simulink model "Galvo_sys_Cdisc_Pcont_cc_nosub_GUT_v63_quantizizer"  (R2013a)
settings: Solver=ode23  StartTime=0.0  StopTime=5e-3  FixedStep=FS  MaxStep=1e-4  RelTol=1e-3
PreLoadFcn:
  | vname=@(x) inputname(1);
  | paramCtrl=evalin('base','paramCtrl;');
  | I_LIM=str2num(paramCtrl.I_LIM);
  | Kbc=str2num(paramCtrl.Kbc);
  | FS=evalin('base','FS;');
InitFcn:
  | %%%%%%  set scope time range
  | T_STOP=str2num(get_param(gcs,'StopTime'));
  | if numel(T_STOP) > 1
  |    T_STOP=T_STOP(2);
  | else
  |    T_STOP=T_STOP(1);
  | end
  | T_STOP=num2str(T_STOP);
  | 
  | %%%%%%  set scope time range in system @init_callback_fct
  | T_STOP=num2str(str2num(get_param(gcs,'StopTime')));
  | 
  | childs = allchild(0);
  | sol=strfind(upper(get(allchild(0),'Tag')),'VIEWER_PARAMETERS');
  | 
  | if iscell(sol)
  |    ind=find(~cellfun(@isempty, strfind(upper(get(allchild(0),'Tag')),'VIEWER_PARAMETERS')));
  | else
  |    ind=sol;
  | end
  | %ind=find(~cellfun(@isempty, {strfind(upper(get(allchild(0),'Tag')),'VIEWER_PARAMETERS'),[]}))
  | if ~isempty(ind)
  |    for k=1:length(childs(ind))
  |       set_param(getfield(get(childs(ind(k)),'UserData'),'block'),'TimeRange',T_STOP);
  |       get_param(getfield(get(childs(ind(k)),'UserData'),'block'),'TimeRange');
  | %    set_param(getfield(get(childs(ind),'UserData'),'block'),'TimeRange',T_STOP);
  | %    get_param(getfield(get(childs(ind),'UserData'),'block'),'TimeRange');
  |    end
  | else
  |     warning(sprintf('VIEWER_PARAMETERS object not found\nOpen the config dialog by hand for the first sim start'))
  | end
StartFcn:
  | I_LIM=str2num(paramCtrl.I_LIM);
  | Kbc=str2num(paramCtrl.Kbc);
  | %FS=evalin('base','FS;');
undefined symbols (not defined in the file or in its folder): FB_EN, JR, KBM, KFR, KMT, KTB, Lc, Rc, Rsh
libraries: simulink x3, simulink_extras x1, dspsigops x1
settings Model: BufferReuse=off  Creator=mainster  LastModifiedBy=mainster
settings SolverCC: AutoInsertRateTranBlk=on
settings DataIOCC: LimitDataPoints=off  SaveOutput=off  SaveTime=off
settings OptimizationCC: BlockReduction=off  OptimizeBlockIOStorage=off  BufferReuse=off  ExpressionFolding=off  LocalBlockOutputs=off
settings ModelReferenceCC: ModelReferenceNumInstancesAllowed=Single

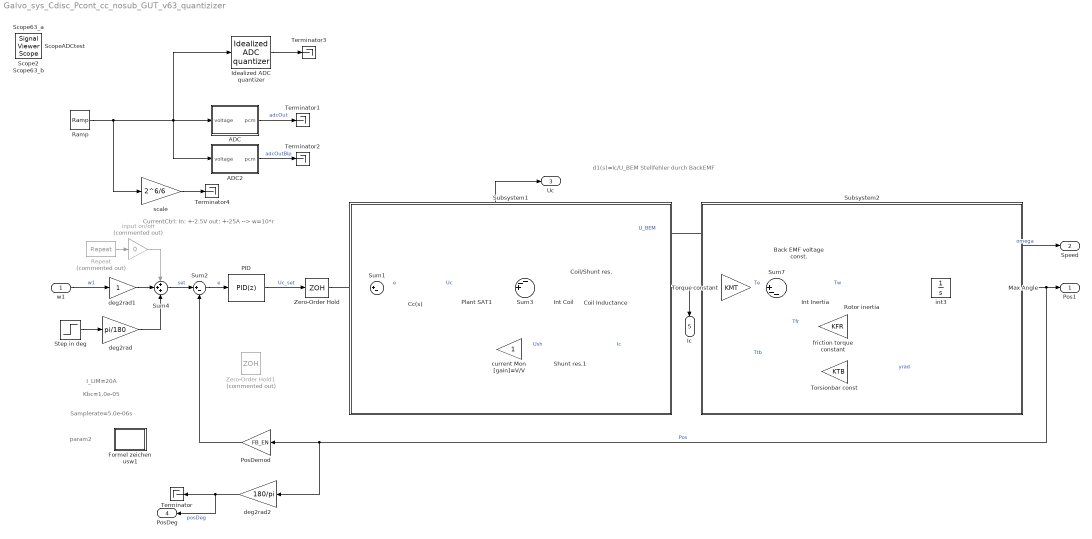
== system Galvo_sys_Cdisc_Pcont_cc_nosub_GUT_v63_quantizizer ==
  note: I_LIM=20A
  note: Kbc=1.0e-05
  note: Samplerate=5.0e-06s
  note: d1(s)=Ic/U_BEM
      | Stellfehler durch BackEMF
  note: param2
  note: CurrentCtrl:
      | In:		+-2.5V
      | out: 	+-25A
      | --> w=10*r
  w1 : Inport
  ADC : Subsystem
      mask Display: fprintf('ADC\n4-bit\n0-3V');
  ADC2 : Subsystem
      mask Display: fprintf('ADC\n4-bit\n-3...+3V');
  Back EMF voltage const. : Gain  Gain=KBM
  Cc(s) : simulink/Continuous/PID Controller  Controller=P  TimeDomain=Continuous-time  SampleTime=-1  IntegratorMethod=Forward Euler  FilterMethod=Forward Euler  Form=Ideal  P=18.7463154861029  I=14078.2261040339  D=0  N=100  InitialConditionSource=internal  InitialConditionForIntegrator=0  InitialConditionForFilter=0  ExternalReset=none  LimitOutput=off  UpperSaturationLimit=inf  LowerSaturationLimit=-inf  LinearizeAsGain=on  AntiWindupMode=none  Kb=1  TrackingMode=off  Kt=1  PParamMin=[]  PParamMax=[]  IParamMin=[]  IParamMax=[]  DParamMin=[]  DParamMax=[]  NParamMin=[]  NParamMax=[]  KbParamMin=[]  KbParamMax=[]  KtParamMin=[]  KtParamMax=[]  POutMin=[]  POutMax=[]  IOutMin=[]  IOutMax=[]  DOutMin=[]  DOutMax=[]  NOutMin=[]  NOutMax=[]  KbOutMin=[]  KbOutMax=[]  KtOutMin=[]  KtOutMax=[]  IntegratorOutMin=[]  IntegratorOutMax=[]  FilterOutMin=[]  FilterOutMax=[]  SumOutMin=[]  SumOutMax=[]  SumI1OutMin=[]  SumI1OutMax=[]  SumI2OutMin=[]  SumI2OutMax=[]  SumI3OutMin=[]  SumI3OutMax=[]  SumDOutMin=[]  SumDOutMax=[]  SaturationOutMin=[]  SaturationOutMax=[]  IntegratorContinuousStateAttributes=''  IntegratorStateMustResolveToSignalObject=off  IntegratorRTWStateStorageClass=Auto  FilterContinuousStateAttributes=''  FilterStateMustResolveToSignalObject=off  FilterRTWStateStorageClass=Auto
  Coil Inductance : Gain  Gain=1/Lc
  Coil/Shunt res. : Gain  Gain=Rc+Rsh
  Formel zeichen usw1 : Subsystem
  Idealized ADC quantizer : simulink_extras/Additional Discrete/Idealized ADC quantizer  NumberOfConverterBits=6  Vmin=-3  Vmax=3  OutputDataType=int16  OutputNegativeValues=on
  Int Coil : Integrator
  Int Inertia : Integrator
  Max Angle : Saturate  UpperLimit=20*pi/180  LowerLimit=-20*pi/180
      settings: AttributesFormatString=Max=%<UpperLimit>\nMin=%<LowerLimit>
  PID : simulink/Continuous/PID Controller  Controller=PID  TimeDomain=Discrete-time  SampleTime=FS  IntegratorMethod=Forward Euler  FilterMethod=Forward Euler  Form=Parallel  P=0.563018062290823  I=5.34105790707236  D=0.011981641194752  N=2584.7602075578  InitialConditionSource=internal  InitialConditionForIntegrator=0  InitialConditionForFilter=0  ExternalReset=none  IgnoreLimit=on  LimitOutput=on  UpperSaturationLimit=30  LowerSaturationLimit=-30  LinearizeAsGain=off  AntiWindupMode=clamping  Kb=0.1  TrackingMode=off  Kt=0  PParamMin=[]  PParamMax=[]  IParamMin=[]  IParamMax=[]  DParamMin=[]  DParamMax=[]  NParamMin=[]  NParamMax=[]  KbParamMin=[]  KbParamMax=[]  KtParamMin=[]  KtParamMax=[]  POutMin=[]  POutMax=[]  IOutMin=[]  IOutMax=[]  DOutMin=[]  DOutMax=[]  NOutMin=[]  NOutMax=[]  KbOutMin=[]  KbOutMax=[]  KtOutMin=[]  KtOutMax=[]  IntegratorOutMin=[]  IntegratorOutMax=[]  FilterOutMin=[]  FilterOutMax=[]  SumOutMin=[]  SumOutMax=[]  SumI1OutMin=[]  SumI1OutMax=[]  SumI2OutMin=[]  SumI2OutMax=[]  SumI3OutMin=[]  SumI3OutMax=[]  SumDOutMin=[]  SumDOutMax=[]  SaturationOutMin=[]  SaturationOutMax=[]  IntegratorContinuousStateAttributes=''  IntegratorStateMustResolveToSignalObject=off  IntegratorRTWStateStorageClass=Auto  FilterContinuousStateAttributes=''  FilterStateMustResolveToSignalObject=off  FilterRTWStateStorageClass=Auto
  Plant SAT1 : Saturate  UpperLimit=30  LowerLimit=-30
      settings: AttributesFormatString=U_lim=+-%<UpperLimit>V
  PosDemod : Gain  Gain=FB_EN
  Ramp : simulink/Sources/Ramp  slope=6/5e-3  start=0  X0=-3
  Repeat : dspsigops/Repeat  Commented=on  N=length(str2num(get_param([gcs '/Sequence Stair'], 'OutValues')))  InputProcessing=Columns as channels (frame based)  RateOptions=Allow multirate processing  ic=0  mode=Unused parameter value
  Rotor inertia : Gain  Gain=1/JR
  Shunt res.1 : Gain
  Step in deg : Step  Time=1e-3  After=5  SampleTime=FS  ZeroCross=off
      settings: AttributesFormatString=Ampl.: %<After>\ntime:%<Time>
  Subsystem1 : Subsystem
      mask Display: text(.05,.05,['{\fontsize{13}\it\bfCurrent comp}'],'horizontalAlignment','left','verticalAlignment','bottom','texmode','on')
  Subsystem2 : Subsystem
      mask Display: text(.05,.05,['{\fontsize{13}\it\bfGalvo mechanic}'],'horizontalAlignment','left','verticalAlignment','bottom','texmode','on')
  Sum1 : Sum  Inputs=|+-
  Sum2 : Sum  Inputs=|+-
  Sum3 : Sum  Inputs=--+||
  Sum4 : Sum  Inputs=+++  SampleTime=FS
  Sum7 : Sum  Inputs=||+--
  Terminator{,1..4} (5 alike) : Terminator
  Torque constant : Gain  Gain=KMT
  Torsionbar const : Gain  Gain=KTB
  Zero-Order Hold : ZeroOrderHold  SampleTime=FS
  Zero-Order Hold1 : ZeroOrderHold  Commented=on  SampleTime=FS
  current Mon [gain]=V/V : Gain
  deg2rad : Gain  Gain=pi/180  SampleTime=FS
  deg2rad1 : Gain  SampleTime=FS
  deg2rad2 : Gain  Gain=180/pi
  friction torque constant : Gain  Gain=KFR
  input on/off : Gain  Commented=on  Gain=0  SampleTime=FS
  int3 : Integrator
  scale : Gain  Gain=2^6/6  SaturateOnIntegerOverflow=on  OutDataTypeStr=Inherit: Same as input  ParamDataTypeStr=Inherit: Same as input
  Pos1 : Outport
  Speed : Outport  Port=2
  Uc : Outport  Port=3
  PosDeg : Outport  Port=4
  Ic : Outport  Port=5
  Scope2 : SignalViewerScope  IOType=viewer  RefreshTime=0.035000
      settings: TickLabels=on  ShowDataMarkers=on  ShowLegends=on  TimeRange=0.0005  YMin=-0.03  YMax=0.065  SaveName=ScopeData2
  Scope63_a : SignalViewerScope  IOType=viewer  NumInputPorts=5  RefreshTime=0.033391
      settings: ShowLegends=on  TimeRange=0.005  YMin=-0.2~-30~-30~-1000~-10  YMax=0.2~30~30~1000~10
  Scope63_b : SignalViewerScope  IOType=viewer  LegendLocations="0.75287     0.88203     0.19598    0.040161"  RefreshTime=0.035000
      settings: ShowLegends=on  TimeRange=0.02  YMin=0  YMax=0.12
  ScopeADCtest : SignalViewerScope  IOType=viewer  NumInputPorts=2  ZoomMode=xonly  RefreshTime=0.035000
      settings: ShowLegends=on  TimeRange=0.005  YMin=-35~-32.5  YMax=30~15  SaveName=ScopeData3
  wires:
  w1/1 -> deg2rad1/1  "w1"
  Repeat/1 -> input on/off/1
  Sum2/1 -> PID/1  "e"
  Sum4/1 -> Sum2/1  "set"
  Step in deg/1 -> deg2rad/1
  input on/off/1 -> Sum4/1
  deg2rad/1 -> Sum4/3
  int3/1 -> Max Angle/1, Torsionbar const/1  "yrad"
  Int Inertia/1 -> Rotor inertia/1  "Tw"
  Sum7/1 -> Int Inertia/1
  Rotor inertia/1 -> Speed/1, int3/1, Back EMF voltage const./1, friction torque constant/1  "omega"
  friction torque constant/1 -> Sum7/3  "Tfr"
  Max Angle/1 -> deg2rad2/1, PosDemod/1, Pos1/1  "Pos"
  Torque constant/1 -> Sum7/1  "Te"
  Torsionbar const/1 -> Sum7/2  "Ttb"
  PID/1 -> Zero-Order Hold/1  "Uc_set"
  deg2rad2/1 -> PosDeg/1, Terminator/1  "posDeg"
  Sum1/1 -> Cc(s)/1  "e"
  Coil Inductance/1 -> Ic/1, Torque constant/1, Shunt res.1/1, Coil/Shunt res./1  "Ic"
  Coil/Shunt res./1 -> Sum3/1
  Sum3/1 -> Int Coil/1
  Int Coil/1 -> Coil Inductance/1
  Cc(s)/1 -> Plant SAT1/1  "Uc"
  Shunt res.1/1 -> current Mon [gain]=V/V/1  "Ush"
  current Mon [gain]=V/V/1 -> Sum1/2
  Plant SAT1/1 -> Uc/1, Sum3/3
  Back EMF voltage const./1 -> Sum3/2  "U_BEM"
  deg2rad1/1 -> Sum4/2
  Zero-Order Hold/1 -> Sum1/1
  PosDemod/1 -> Sum2/2
  ADC/1(pcm) -> Terminator1/1  "adcOut"
  ADC2/1(pcm) -> Terminator2/1  "adcOutBip"
  Idealized ADC quantizer/1 -> Terminator3/1
  Ramp/1 -> scale/1, Idealized ADC quantizer/1, ADC2/1(voltage), ADC/1(voltage)
  scale/1 -> Terminator4/1

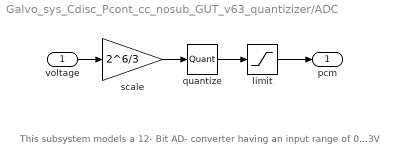
== system Galvo_sys_Cdisc_Pcont_cc_nosub_GUT_v63_quantizizer/ADC ==
  note: This subsystem models a 12- Bit AD- converter
      | having an input  range of 0...3V
  voltage : Inport
  limit : Saturate  UpperLimit=2^12  LowerLimit=0
  quantize : Quantizer
  scale : Gain  Gain=2^6/3  SaturateOnIntegerOverflow=on  OutDataTypeStr=Inherit: Same as input  ParamDataTypeStr=Inherit: Same as input
  pcm : Outport
  wires:
  limit/1 -> pcm/1
  scale/1 -> quantize/1
  quantize/1 -> limit/1
  voltage/1 -> scale/1

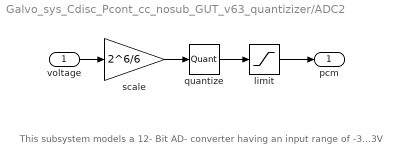
== system Galvo_sys_Cdisc_Pcont_cc_nosub_GUT_v63_quantizizer/ADC2 ==
  note: This subsystem models a 12- Bit AD- converter
      | having an input  range of -3...3V
  voltage : Inport
  limit : Saturate  UpperLimit=2^5-1  LowerLimit=-2^5
  quantize : Quantizer
  scale : Gain  Gain=2^6/6  SaturateOnIntegerOverflow=on  OutDataTypeStr=Inherit: Same as input  ParamDataTypeStr=Inherit: Same as input
  pcm : Outport
  wires:
  limit/1 -> pcm/1
  scale/1 -> quantize/1
  quantize/1 -> limit/1
  voltage/1 -> scale/1

== system Galvo_sys_Cdisc_Pcont_cc_nosub_GUT_v63_quantizizer/Formel zeichen usw1 ==
  note: Te: 		electrical torque, gen. by coils		[Nm]
      |  Ic: 			coil current							[A]
      |  Tfr:		rotor dynamic friction torque 		[Nm]
      |  Trb:		torsion bar torque					[Nm]
      |  Tw:		angular momentum				[Nm*s]
      |  w:			angular velocity 					[rad/s]
      |  yrad:		angular position 					[rad]
      |  ydeg:		angular position 					[°]
      |  Ucci:		current controller input				[V]
      |  Ucco:		current controller output			[V]
      |  Ush:		shunt voltage						[V]
  note: L_{c  }	coil inductance 							[H]
      |  R_{c  }	coil resistance							[\Omega]
      |  R_{SH }	current shunt resistance				[\Omega]
      |  J_{R  }	rotor inertia 							[kg*m²]
      |  K_{TB }	torsion bar torque const. 			[Nm/rad]
      |  K_{BM }	back EMF const.							[V*s/rad]
      |  K_{FR }	rotor dyn. friction torque const.	[Nm*s/rad]
      |  K_{MT }	el. magnetic torque const.			[Nm/A]
  note: balance of force: 	Te=Ttb+Tfr
      | 					Te - (Ttb+Tfr)=0  ->  no movement
      |
      |  integrate( 1 Nm )dt = 1 Nm*s
      |  (Nm*s)(kg*m²)⁻¹ = (N*s/kg)*m⁻¹ = m/(s*m) = rad

== system Galvo_sys_Cdisc_Pcont_cc_nosub_GUT_v63_quantizizer/Subsystem1 ==

== system Galvo_sys_Cdisc_Pcont_cc_nosub_GUT_v63_quantizizer/Subsystem2 ==
